simulink subsystem "LaneMetrics"  (R2024b)
settings: Solver=VariableStepAuto  StartTime=0.0  StopTime=10.0  RelTol=1e-3
undefined symbols (not defined in the file or in its folder): camera
libraries: simulink x2
settings Model: Creator=The MathWorks, Inc.  LastModifiedBy=The MathWorks, Inc.
settings SolverCC: MaxZcPerStep=1
settings OptimizationCC: ReuseModelBlockBuffer=off
settings DebuggingCC: UnconnectedInputMsg=warning  UnconnectedOutputMsg=warning  UnconnectedLineMsg=warning  SubsystemReferenceDiagnosticForUnitTest=warning
settings ModelReferenceCC: EnableRefExpFcnMdlSchedulingChecks=on
settings RTWCC: GPUComputeCapability=3.5  DLArmComputeVersion=19.05

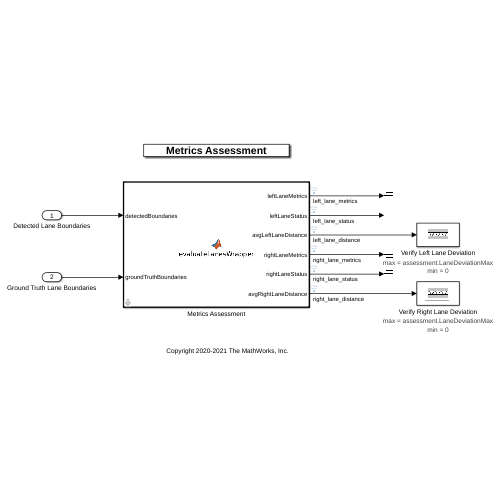
[thumbnail: Simulink's stored preview of the top-level diagram]
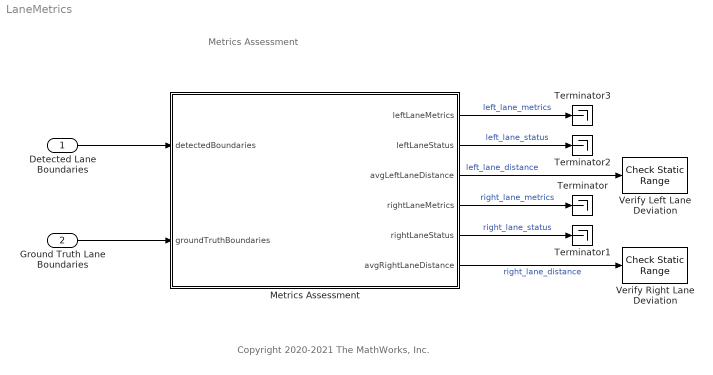
== system LaneMetrics ==
  note: Metrics Assessment
  note: Copyright 2020-2021 The MathWorks, Inc.
  Detected Lane Boundaries : Inport
  Ground Truth Lane Boundaries : Inport  Port=2
  Metrics Assessment : MATLAB Function  TreatAsAtomicUnit=on  mask{detectionRange=camera.LaneDetectionRanges}
      mask prompts: detectionRange "Lane Assessment Range"
  Terminator{,1..3} (4 alike) : Terminator
  Verify Left Lane Deviation : simulink/Model Verification/Check  Static Range  Description=0 <= u <= assessment.LaneDeviationMax  max=assessment.LaneDeviationMax  max_included=on  min=0  min_included=on  enabled=on  stopWhenAssertionFail=off  export=off  icon=graphic
      settings: AttributesFormatString=|
      | max = %<max>
      | min = %<min>
  Verify Right Lane Deviation : simulink/Model Verification/Check  Static Range  Description=0 <= u <= assessment.LaneDeviationMax  max=assessment.LaneDeviationMax  max_included=on  min=0  min_included=on  enabled=on  stopWhenAssertionFail=off  export=off  icon=graphic
      settings: AttributesFormatString=|
      | max = %<max>
      | min = %<min>
  wires:
  Metrics Assessment/1(leftLaneMetrics) -> Terminator3/1  "left_lane_metrics"
  Ground Truth Lane Boundaries/1 -> Metrics Assessment/2(groundTruthBoundaries)
  Detected Lane Boundaries/1 -> Metrics Assessment/1(detectedBoundaries)
  Metrics Assessment/4(rightLaneMetrics) -> Terminator/1  "right_lane_metrics"
  Metrics Assessment/3(avgLeftLaneDistance) -> Verify Left Lane Deviation/1  "left_lane_distance"
  Metrics Assessment/5(rightLaneStatus) -> Terminator1/1  "right_lane_status"
  Metrics Assessment/6(avgRightLaneDistance) -> Verify Right Lane Deviation/1  "right_lane_distance"
  Metrics Assessment/2(leftLaneStatus) -> Terminator2/1  "left_lane_status"

== matlab function LaneMetrics/Metrics Assessment ==
  data: detectedBoundaries input; groundTruthBoundaries input; detectionRange parameter; leftLaneMetrics output; leftLaneStatus output; avgLeftLaneDistance output; rightLaneMetrics output; rightLaneStatus output; avgRightLaneDistance output
function [leftLaneMetrics,leftLaneStatus,avgLeftLaneDistance,...
    rightLaneMetrics,rightLaneStatus,avgRightLaneDistance ] = ...
    evaluateLanesWrapper(detectedBoundaries, groundTruthBoundaries, detectionRange)

leftLaneMetrics  = zeros(1,3);
leftLaneStatus = 0;
avgLeftLaneDistance = 0;
rightLaneMetrics = zeros(1,3); 
rightLaneStatus  = 0;
avgRightLaneDistance = 0;

coder.extrinsic('helperComputeLaneMetrics');

[leftLaneMetrics, leftLaneStatus, avgLeftLaneDistance,...
    rightLaneMetrics, rightLaneStatus, avgRightLaneDistance ] = ...
    helperComputeLaneMetrics(detectedBoundaries,groundTruthBoundaries, detectionRange);
end
